simulink model "pmsm_Linear_ssModel_3P_nocontroller"  (R2024a)
settings: Solver=VariableStepAuto  StartTime=0.0  StopTime=100  RelTol=1e-3
values from neighbouring files (symbols this model uses):
  A = 2 * R_circle * dot(d_vec, u_vec)    [full_3d_suspension_dashboard_pro11.m]
  B = 2 * R_circle * dot(d_vec, v_vec)    [full_3d_suspension_dashboard_pro11.m]
  C = [0, C_y, C_z]    [full_3d_suspension_dashboard_pro11.m]
  D = [0, D_y, D_z]    [full_3d_suspension_dashboard_pro11.m]
settings Model: Creator=Vaibhav Inamdar  LastModifiedBy=Vaibhav Inamdar
settings ConfigComp: CovBoundaryAbsTol=1.0e-5

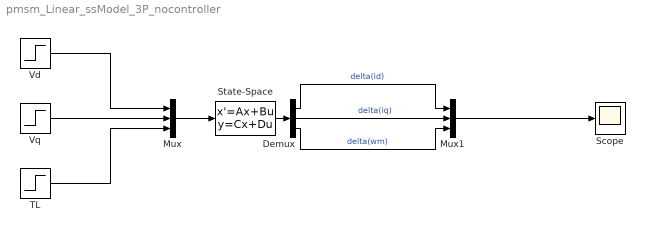
== system pmsm_Linear_ssModel_3P_nocontroller ==
  Demux : Demux  Outputs=3
  Mux : Mux  Inputs=3
  Mux1 : Mux  Inputs=3
  Scope : Scope
  State-Space : StateSpace  A=A  B=B  C=C  D=D  InitialCondition=0
  TL : Step  Time=0  After=0  SampleTime=0
  Vd : Step  Time=0  After=0  SampleTime=0
  Vq : Step  Time=0  After=5  SampleTime=0
  wires:
  Mux/1 -> State-Space/1
  Vd/1 -> Mux/1
  TL/1 -> Mux/3
  State-Space/1 -> Demux/1
  Demux/1 -> Mux1/1  "delta(id)"
  Demux/2 -> Mux1/2  "delta(iq)"
  Mux1/1 -> Scope/1
  Demux/3 -> Mux1/3  "delta(wm)"
  Vq/1 -> Mux/2
